simulink model "bh_test_obsv"  (R2021a)
settings: Solver=ode15s  StartTime=0.0  StopTime=10  FixedStep=0.0005  RelTol=1e-5
undefined symbols (not defined in the file): Continuous, Time
libraries: cstblocks x2, ctrlSharedLib x1
settings Model: Creator=bhorton  LastModifiedBy=bhorton
settings SolverCC: ZeroCrossAlgorithm=Adaptive
settings ExplorerConfigSet: InternalSimMechanicsExplorerSettings="<ExplorerConfiguration><canonicalview>default</canonicalview><AnimationSetting><BasePlaybackSpeed>1.0</BasePlaybackSpeed><PlaybackSpeedFactor>1.0</PlaybackSpeedFactor></AnimationSetting><TilePanel><TileInfo><Tiles Columns=\"2\" Count=\"3\" Rows=\"2\"><Column Weight=\"0.4994\"/><Column Weight=\"0.5006\"/><Row Weight=\"0.4993\"/><Row Weight=\"0.5007\"/><Tile Height=\"1\" Width=\"2\" X=\"0\" Y=\"0\"/><Tile Height=\"1\" Width=\"1\" X=\"0\" Y=\"1\"/><Tile Height=\"1\" Width=\"1\" X=\"1\" Y=\"1\"/></Tiles></TileInfo><SceneInfo><SceneViewer><BGColor><R>0.60000002384185791</R><G>0.60000002384185791</G><B>0.60000002384185791</B></BGColor><Camera><DoPerspective>off</DoPerspective><Position><X>21.8610799900497348</X><Y>10.2157712548228687</Y><Z>27.1304269960658964</Z></Position><Center><X>2.57683900679416</X><Y>1.27770136551759128</Y><Z>-0.515230289296268573</Z></Center><Up><X>-0.185673330126828295</X><Y>0.96548958646651295</Y><Z>-0.182634259941381938</Z></Up><ViewLimDist>1</ViewLimDist><YLim>2.25822710766344814</YLim><XLim>8.49645176480614062</XLim></Camera></SceneViewer><SceneViewer><BGColor><R>0.60000002384185791</R><G>0.60000002384185791</G><B>0.60000002384185791</B></BGColor><Camera><DoPerspective>off</DoPerspective><Position><X>5.56922306449081894</X><Y>11.1809852242994197</Y><Z>70.2283409642136576</Z></Position><Center><X>1.69410129434751933</X><Y>1.57692293746242651</Y><Z>-0.880736604599208439</Z></Center><Up><X>-0.0228131350943184333</X><Y>0.990908416802929626</Y><Z>-0.132589857742894418</Z></Up><ViewLimDist>1</ViewLimDist><YLim>1.61301502827887266</YLim><XLim>3.00078921927556053</XLim></Camera></SceneViewer><SceneViewer><BGColor><R>0.60000002384185791</R><G>0.60000002384185791</G><B>0.60000002384185791</B></BGColor><Camera><DoPerspective>off</DoPerspective><Position><X>16.4092255072445212</X><Y>2.30299630530687338</Y><Z>-1.68120805435522325</Z></Position><Center><X>1.71666123588749886</X><Y>0.68646529793520239</Y><Z>-2.57293573701102085</Z></Center><Up><X>-0.109797444713875203</X><Y>0.993927323497863835</Y><Z>0.0072798858972461869</Z></Up><ViewLimDist>1</ViewLimDist><YLim>1.82496821621514438</YLim><XLim>3.40331910591472875</XLim></Camera></SceneViewer></SceneInfo></TilePanel><MechEditorPanel><Cameras/><GfxPanelCameraMap/><VideoCreator><PlaybackSpeedRatio>1.0</PlaybackSpeedRatio><FrameRate>30</FrameRate><VideoFormat>MPEG-4</VideoFormat><FrameSize>[400 400]</FrameSize></VideoCreator></MechEditorPanel></ExplorerConfiguration>"

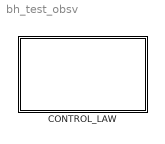
== system bh_test_obsv ==
  CONTROL_LAW : Subsystem

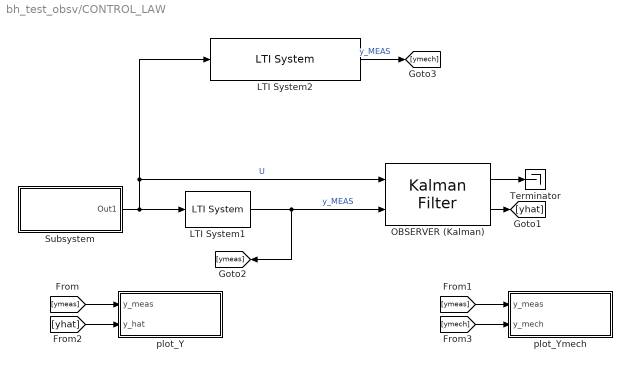
== system bh_test_obsv/CONTROL_LAW ==
  LTI System1 : cstblocks/LTI System  sys=my_sys  IC=[]
  LTI System2 : cstblocks/LTI System  sys=my_ss_MECH_sys  IC=[]
  OBSERVER (Kalman) : ctrlSharedLib/Kalman Filter  TimeDomain=Continuous-Time  UseCurrentEstimator=on  ModelSource=LTI State-Space Variable  ModelSourceVariable=my_sys  A=0.95  B=1  C=1  D=0  NumberOfStates=1  NumberOfInputs=1  NumberOfOutputs=1  InitialEstimateSource=Dialog  X0=0  P0=10  UseK=off  UseGH=off  NumberOfProcessNoiseInputs=1  G=1  TimeInvariantG=on  H=0  TimeInvariantH=on  Q=1e8  TimeInvariantQ=on  R=1  TimeInvariantR=on  N=0  TimeInvariantN=on  AddInputPort=on  AddEnablePort=off  OutputEstimatedY=on  OutputP=off  Ts=-1
  Subsystem : Subsystem
  Terminator : Terminator
  plot_Y : Subsystem
  plot_Ymech : Subsystem
  wires:
  LTI System1/1 -> OBSERVER (Kalman)/2, [ymeas]  "y_MEAS"
  OBSERVER (Kalman)/2 -> [yhat]
  [ymeas] -> plot_Y/1(y_meas)
  [yhat] -> plot_Y/2(y_hat)
  Subsystem/1(Out1) -> LTI System2/1, OBSERVER (Kalman)/1, LTI System1/1  "U"
  OBSERVER (Kalman)/1 -> Terminator/1
  LTI System2/1 -> [ymech]  "y_MEAS"
  [ymeas] -> plot_Ymech/1(y_meas)
  [ymech] -> plot_Ymech/2(y_mech)

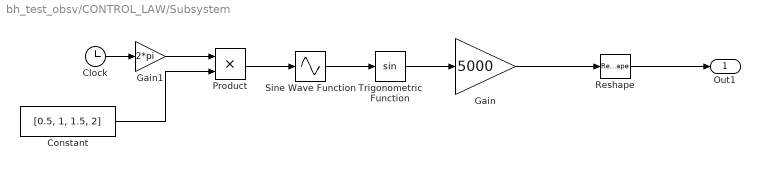
== system bh_test_obsv/CONTROL_LAW/Subsystem ==
  Clock : Clock
  Constant : Constant  Value=[0.5, 1, 1.5, 2]
  Gain : Gain  Gain=5000
  Gain1 : Gain  Gain=2*pi
  Product : Product
  Reshape : Reshape  OutputDimensionality=Column vector (2-D)
  Sine Wave Function : Sin  TimeSource=Use external signal  SampleTime=0
  Trigonometric Function : Trigonometry
  Out1 : Outport
  wires:
  Clock/1 -> Gain1/1
  Constant/1 -> Product/2
  Gain1/1 -> Product/1
  Product/1 -> Sine Wave Function/1
  Sine Wave Function/1 -> Trigonometric Function/1
  Trigonometric Function/1 -> Gain/1
  Gain/1 -> Reshape/1
  Reshape/1 -> Out1/1

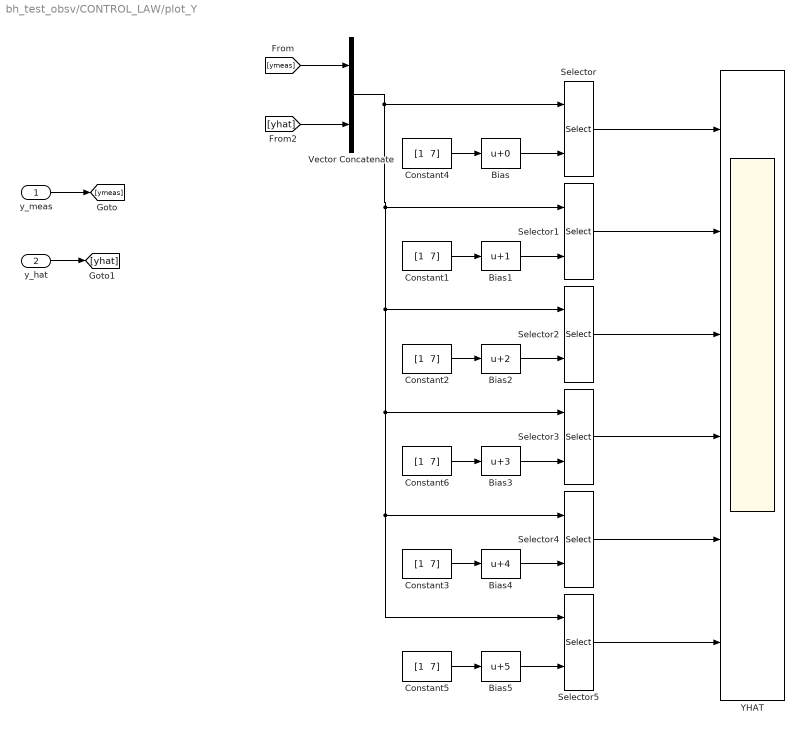
== system bh_test_obsv/CONTROL_LAW/plot_Y ==
  y_meas : Inport
  y_hat : Inport  Port=2
  Bias : Bias
  Bias1 : Bias  Bias=1
  Bias2 : Bias  Bias=2
  Bias3 : Bias  Bias=3
  Bias4 : Bias  Bias=4
  Bias5 : Bias  Bias=5
  Constant{1..6} (6 alike) : Constant  Value="[1  7]"
  Selector{,1..5} (6 alike) : Selector  InputPortWidth=12  IndexOptions=Index vector (port)  Indices=[1 3]  OutputSizes=1
  Vector Concatenate : Concatenate
  YHAT : Scope  NumInputPorts=6
  wires:
  y_meas/1 -> [ymeas]
  y_hat/1 -> [yhat]
  [ymeas] -> Vector Concatenate/1
  [yhat] -> Vector Concatenate/2
  Constant4/1 -> Bias/1
  Bias/1 -> Selector/2
  Selector/1 -> YHAT/1
  Bias1/1 -> Selector1/2
  Constant1/1 -> Bias1/1
  Selector1/1 -> YHAT/2
  Bias2/1 -> Selector2/2
  Constant2/1 -> Bias2/1
  Selector2/1 -> YHAT/3
  Bias3/1 -> Selector3/2
  Constant3/1 -> Bias4/1
  Bias4/1 -> Selector4/2
  Vector Concatenate/1 -> Selector3/1, Selector5/1, Selector4/1, Selector2/1, Selector1/1, Selector/1
  Constant6/1 -> Bias3/1
  Bias5/1 -> Selector5/2
  Constant5/1 -> Bias5/1
  Selector3/1 -> YHAT/4
  Selector4/1 -> YHAT/5
  Selector5/1 -> YHAT/6

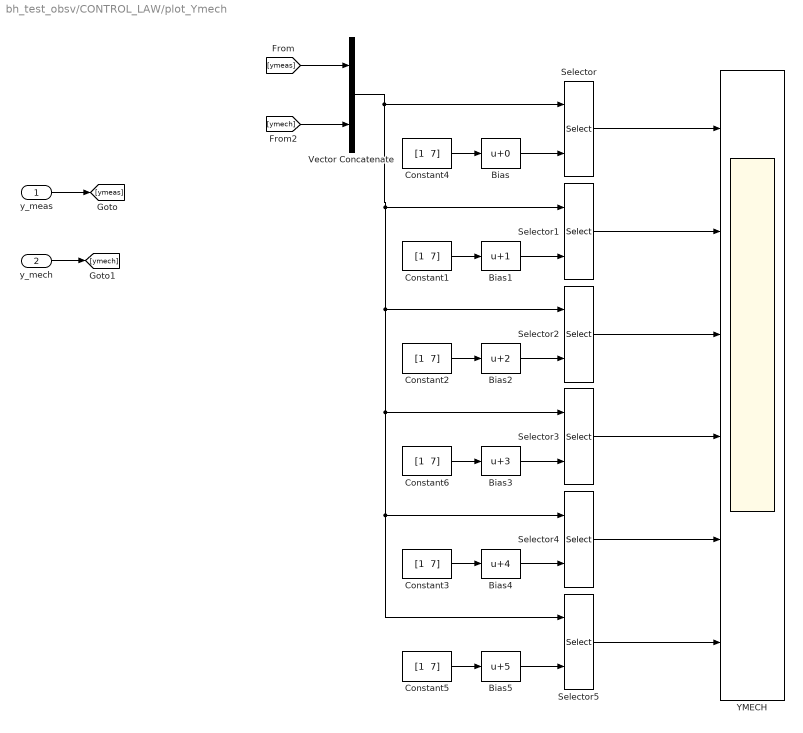
== system bh_test_obsv/CONTROL_LAW/plot_Ymech ==
  y_meas : Inport
  y_mech : Inport  Port=2
  Bias : Bias
  Bias1 : Bias  Bias=1
  Bias2 : Bias  Bias=2
  Bias3 : Bias  Bias=3
  Bias4 : Bias  Bias=4
  Bias5 : Bias  Bias=5
  Constant{1..6} (6 alike) : Constant  Value="[1  7]"
  Selector{,1..5} (6 alike) : Selector  InputPortWidth=12  IndexOptions=Index vector (port)  Indices=[1 3]  OutputSizes=1
  Vector Concatenate : Concatenate
  YMECH : Scope  NumInputPorts=6
  wires:
  y_meas/1 -> [ymeas]
  y_mech/1 -> [ymech]
  [ymeas] -> Vector Concatenate/1
  [ymech] -> Vector Concatenate/2
  Constant4/1 -> Bias/1
  Bias/1 -> Selector/2
  Selector/1 -> YMECH/1
  Bias1/1 -> Selector1/2
  Constant1/1 -> Bias1/1
  Selector1/1 -> YMECH/2
  Bias2/1 -> Selector2/2
  Constant2/1 -> Bias2/1
  Selector2/1 -> YMECH/3
  Bias3/1 -> Selector3/2
  Constant3/1 -> Bias4/1
  Bias4/1 -> Selector4/2
  Vector Concatenate/1 -> Selector3/1, Selector5/1, Selector4/1, Selector2/1, Selector1/1, Selector/1
  Constant6/1 -> Bias3/1
  Bias5/1 -> Selector5/2
  Constant5/1 -> Bias5/1
  Selector3/1 -> YMECH/4
  Selector4/1 -> YMECH/5
  Selector5/1 -> YMECH/6
